simulink model "carBalance"  (R2019a)
settings: Solver=VariableStepAuto  StartTime=0.0  StopTime=10.0  RelTol=1e-3
values from neighbouring files (symbols this model uses):
  a1 = A(1)    [test.m]
  a10 = B(5)    [test.m]
  a2 = A(2)    [test.m]
  a3 = A(3)    [test.m]
  a4 = A(4)    [test.m]
  a5 = A(5)    [test.m]
  a6 = B(1)    [test.m]
  a7 = B(2)    [test.m]
  a8 = B(3)    [test.m]
  a9 = B(4)    [test.m]
undefined symbols (not defined in the file or in its folder): DiscIntNeverNeededParam
settings Model: Creator=USER  LastModifiedBy=USER

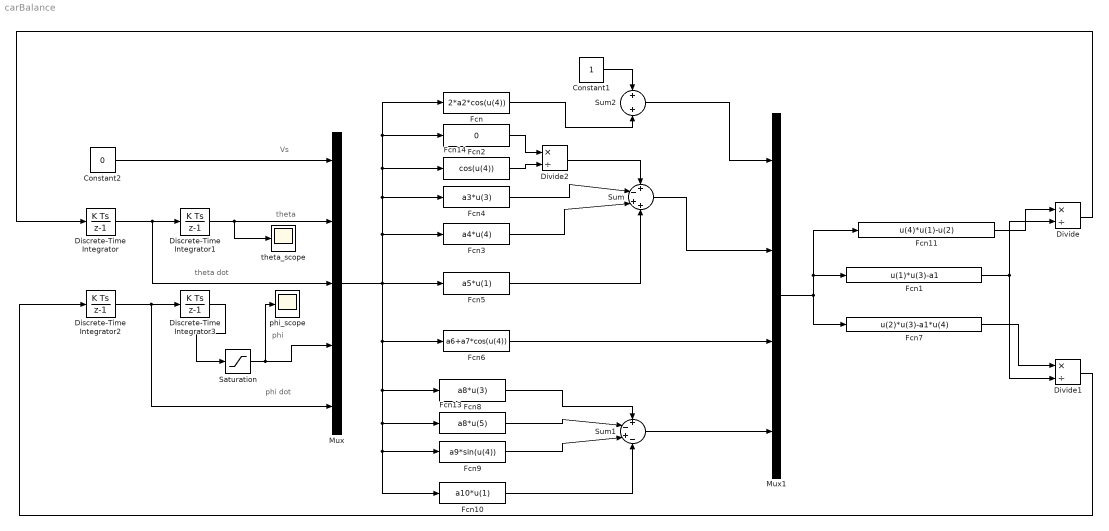
== system carBalance ==
  note: phi dot
  note: theta
  note: phi
  note: Vs
  note: theta dot
  Constant1 : Constant
  Constant2 : Constant  Value=0
  Discrete-Time Integrator : DiscreteIntegrator  SampleTime=0.0001  ICPrevOutput=DiscIntNeverNeededParam  ICPrevScaledInput=DiscIntNeverNeededParam
  Discrete-Time Integrator1 : DiscreteIntegrator  SampleTime=0.0001  ICPrevOutput=DiscIntNeverNeededParam  ICPrevScaledInput=DiscIntNeverNeededParam
  Discrete-Time Integrator2 : DiscreteIntegrator  SampleTime=0.0001  ICPrevOutput=DiscIntNeverNeededParam  ICPrevScaledInput=DiscIntNeverNeededParam
  Discrete-Time Integrator3 : DiscreteIntegrator  InitialCondition=pi/180  SampleTime=0.0001  ICPrevOutput=DiscIntNeverNeededParam  ICPrevScaledInput=DiscIntNeverNeededParam
  Divide : Product  Inputs=*/
  Divide1 : Product  Inputs=*/
  Divide2 : Product  Inputs=*/
  Fcn : Fcn  Expr=2*a2*cos(u(4))
  Fcn1 : Fcn  Expr=u(1)*u(3)-a1
  Fcn10 : Fcn  Expr=a10*u(1)
  Fcn11 : Fcn  Expr=u(4)*u(1)-u(2)
  Fcn13 : Fcn  Expr=a8*u(5)
  Fcn14 : Fcn  Expr=cos(u(4))
  Fcn2 : Fcn  Expr=0
  Fcn3 : Fcn  Expr=a4*u(4)
  Fcn4 : Fcn  Expr=a3*u(3)
  Fcn5 : Fcn  Expr=a5*u(1)
  Fcn6 : Fcn  Expr=a6+a7*cos(u(4))
  Fcn7 : Fcn  Expr=u(2)*u(3)-a1*u(4)
  Fcn8 : Fcn  Expr=a8*u(3)
  Fcn9 : Fcn  Expr=a9*sin(u(4))
  Mux : Mux  Inputs=5
  Mux1 : Mux
  Saturation : Saturate  UpperLimit=1.57  LowerLimit=-1.57
  Sum : Sum  Inputs=+-++
  Sum1 : Sum  Inputs=+-+-
  Sum2 : Sum
  "phi_scope " : Scope
  theta_scope : Scope
  wires:
  Fcn6/1 -> Mux1/3
  Discrete-Time Integrator/1 -> Mux/3, Discrete-Time Integrator1/1
  Constant2/1 -> Mux/1
  Discrete-Time Integrator2/1 -> Mux/5, Discrete-Time Integrator3/1
  Fcn8/1 -> Sum1/1
  Sum1/1 -> Mux1/4
  Discrete-Time Integrator3/1 -> Saturation/1
  Saturation/1 -> "phi_scope "/1, Mux/4
  Sum/1 -> Mux1/2
  Fcn3/1 -> Sum/3
  Divide1/1 -> Discrete-Time Integrator2/1
  Discrete-Time Integrator1/1 -> Mux/2, theta_scope/1
  Divide/1 -> Discrete-Time Integrator/1
  Fcn5/1 -> Sum/4
  Fcn4/1 -> Sum/2
  Fcn/1 -> Sum2/2
  Constant1/1 -> Sum2/1
  Sum2/1 -> Mux1/1
  Mux/1 -> Fcn5/1, Fcn6/1, Fcn13/1, Fcn10/1, Fcn9/1, Fcn8/1, Fcn14/1, Fcn2/1, Fcn/1, Fcn4/1, Fcn3/1
  Fcn13/1 -> Sum1/2
  Fcn9/1 -> Sum1/3
  Fcn10/1 -> Sum1/4
  Fcn2/1 -> Divide2/1
  Fcn14/1 -> Divide2/2
  Divide2/1 -> Sum/1
  Mux1/1 -> Fcn11/1, Fcn1/1, Fcn7/1
  Fcn11/1 -> Divide/1
  Fcn1/1 -> Divide/2, Divide1/2
  Fcn7/1 -> Divide1/1
